simulink model "Dynamic_Pressure"  (R2018a)
settings: Solver=VariableStepAuto  StartTime=0.0  StopTime=10.0  RelTol=1e-3
libraries: aerolibasang x1, aerolibatmos2 x1
settings Model: Creator=McQueen_Zero  LastModifiedBy=McQueen_Zero

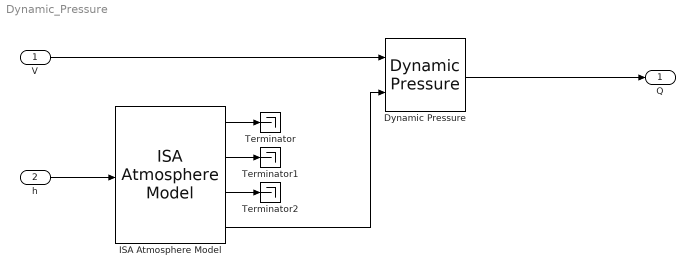
== system Dynamic_Pressure ==
  V : Inport
  h : Inport  Port=2
  Dynamic Pressure : aerolibasang/Dynamic Pressure
  ISA Atmosphere Model : aerolibatmos2/ISA Atmosphere Model  custom=off  g=9.80665  gamma=1.4  R=287.0531  L=0.0065  h_trop=11000  h_strat=20000  rho0=1.225  P0=101325  T0=288.15  h0=0
      settings: SourceProductName=Aerospace Blockset
  Terminator : Terminator
  Terminator1 : Terminator
  Terminator2 : Terminator
  Q : Outport
  wires:
  V/1 -> Dynamic Pressure/1
  Dynamic Pressure/1 -> Q/1
  ISA Atmosphere Model/4 -> Dynamic Pressure/2
  h/1 -> ISA Atmosphere Model/1
  ISA Atmosphere Model/1 -> Terminator/1
  ISA Atmosphere Model/2 -> Terminator1/1
  ISA Atmosphere Model/3 -> Terminator2/1
